simulink model "steer_by_wire"  (R2023b)
settings: Solver=VariableStepAuto  StartTime=0.0  StopTime=10.0  RelTol=1e-3
settings Model: Creator=jcm52  LastModifiedBy=jcm52

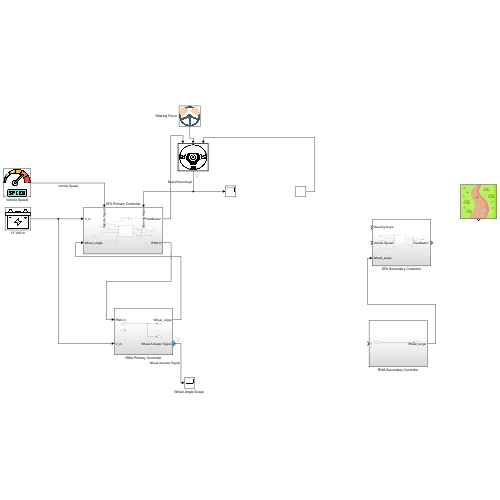
[thumbnail: Simulink's stored preview of the top-level diagram]
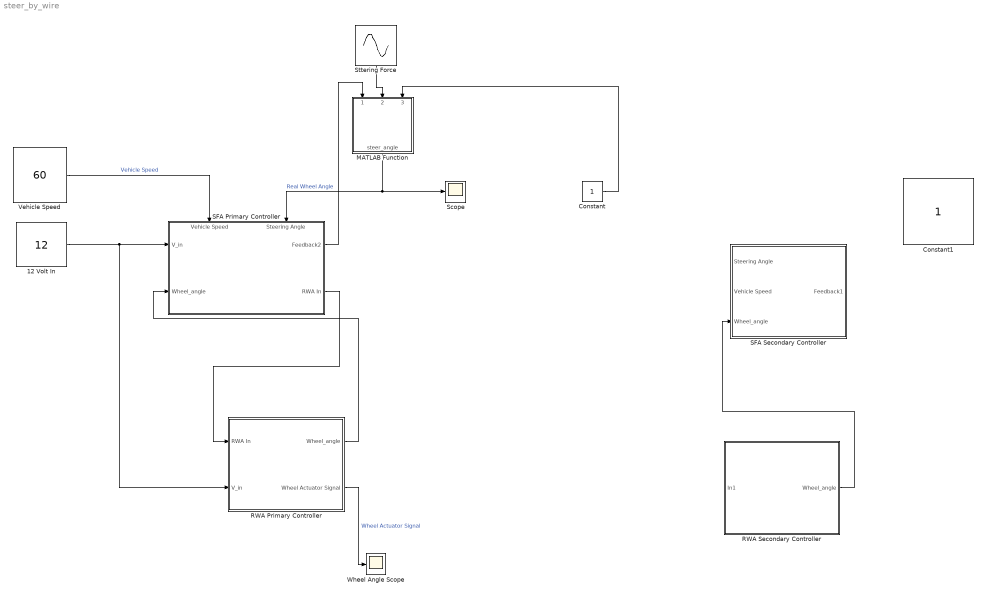
== system steer_by_wire ==
  12 Volt In : Constant  Value=12
      mask Display: image('image\free-icon-battery-3444043.png');
  Constant : Constant
  Constant1 : Constant
      mask Display: image('image\free-icon-footpath-6858832.png');
  MATLAB Function : MATLAB Function  TreatAsAtomicUnit=on
  RWA Primary Controller : Subsystem
  RWA Secondary Controller : Subsystem
  SFA Primary Controller : Subsystem
      settings: PortSchema="{\"entries\":[{\"content\":{\"sides\":[{\"content\":{\"connectorIds\":[\"Out1\",\"Out2\"]},\"type\":\"ConnectorPlacement.EquallySpacedRectSide\",\"uuid\":\"69d6b4e8-6a6c-440e-b630-8ac486e35eae\"},{\"content\":{\"connectorIds\":[\"In3\",\"In4\"],\"side\":\"RIGHT\"},\"type\":\"ConnectorPlacement.EquallySpacedRectSide\",\"uuid\":\"56fbaa10-ad34-420d-babb-7be934bb8fcf\"},{\"content\":{\"connectorIds\":[\"In1\",\"In2\"],\"side\":\"TOP\"},\"type\":\"ConnectorPlacement.EquallySpacedRectSide\",\"uuid\":\"184d897f-af35-4327-bbad-019fb4f06789\"},{\"content\":{\"side\":\"BOTTOM\"},\"type\":\"ConnectorPlacement.EquallySpacedRectSide\",\"uuid\":\"33f7de2b-e358-4395-9aa5-bc9b031e2917\"}]},\"type\":\"ConnectorPlacement.EquallySpacedConnector\",\"uuid\":\"8508fc02-ca2d-4db9-a320-47449abdf9d8\"}],\"packageUris\":[\"http://schema.mathworks.com/mf0/Connector/R2020b\"],\"version\":\"1.0\"}"
  SFA Secondary Controller : Subsystem
  Scope : Scope
  Sttering Force : Sin  Amplitude=180  SampleTime=0
      mask Display: image('image\free-icon-steering-wheel-2297514.png');
  Vehicle Speed : Constant  Value=60
      mask Display: image('image\free-icon-speed-1455318.png');
  "Wheel Angle Scope " : Scope
  wires:
  MATLAB Function/1(steer_angle) -> SFA Primary Controller/1(Steering Angle), Scope/1  "Real Wheel Angle"
  Sttering Force/1 -> MATLAB Function/2(driver_force)
  SFA Primary Controller/1("Feedback2 ") -> MATLAB Function/1(feedback1)
  Vehicle Speed/1 -> SFA Primary Controller/2(Vehicle Speed)  "Vehicle Speed"
  RWA Secondary Controller/1(Wheel_angle) -> SFA Secondary Controller/3(Wheel_angle)
  RWA Primary Controller/1(Wheel_angle) -> SFA Primary Controller/4(Wheel_angle)
  RWA Primary Controller/2(Wheel Actuator Signal) -> "Wheel Angle Scope "/1  "Wheel Actuator Signal"
  12 Volt In/1 -> RWA Primary Controller/2(V_in), SFA Primary Controller/3(V_in)
  SFA Primary Controller/2(RWA In) -> RWA Primary Controller/1(RWA In)
  Constant/1 -> MATLAB Function/3(feedback2)

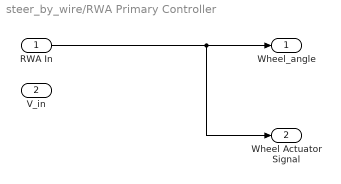
== system steer_by_wire/RWA Primary Controller ==
  RWA In : Inport
  V_in : Inport  Port=2
  Wheel_angle : Outport
  Wheel Actuator Signal : Outport  Port=2
  wires:
  RWA In/1 -> Wheel Actuator Signal/1, Wheel_angle/1

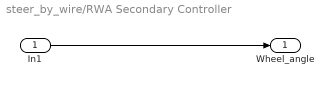
== system steer_by_wire/RWA Secondary Controller ==
  In1 : Inport
  Wheel_angle : Outport
  wires:
  In1/1 -> Wheel_angle/1

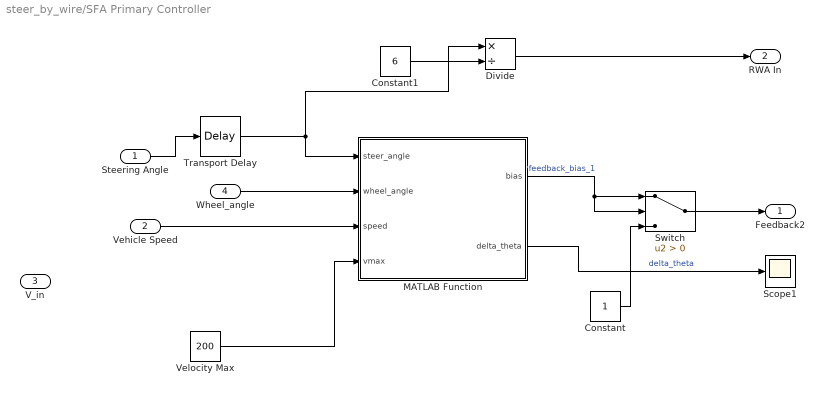
== system steer_by_wire/SFA Primary Controller ==
  Steering Angle : Inport
  Vehicle Speed : Inport  Port=2
  V_in : Inport  Port=3
  Wheel_angle : Inport  Port=4
  Constant : Constant
  Constant1 : Constant  Value=6
  Divide : Product  Inputs=*/
  MATLAB Function : MATLAB Function  TreatAsAtomicUnit=on
  Scope1 : Scope
  Switch : Switch  Criteria=u2 > Threshold  SaturateOnIntegerOverflow=off  InputSameDT=off
  Transport Delay : TransportDelay  DelayTime=0.1
  Velocity Max : Constant  Value=200
  "Feedback2 " : Outport
  RWA In : Outport  Port=2
  wires:
  Constant/1 -> Switch/3
  Switch/1 -> "Feedback2 "/1
  Steering Angle/1 -> Transport Delay/1
  Vehicle Speed/1 -> MATLAB Function/3(speed)
  Wheel_angle/1 -> MATLAB Function/2(wheel_angle)
  Velocity Max/1 -> MATLAB Function/4(vmax)
  MATLAB Function/1(bias) -> Switch/1, Switch/2  "feedback_bias_1"
  Constant1/1 -> Divide/2
  Divide/1 -> RWA In/1
  MATLAB Function/2(delta_theta) -> Scope1/1  "delta_theta"
  Transport Delay/1 -> MATLAB Function/1(steer_angle), Divide/1

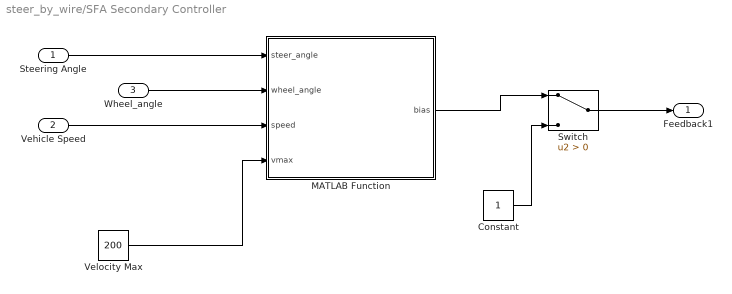
== system steer_by_wire/SFA Secondary Controller ==
  Steering Angle : Inport
  Vehicle Speed : Inport  Port=2
  Wheel_angle : Inport  Port=3
  Constant : Constant
  MATLAB Function : MATLAB Function  TreatAsAtomicUnit=on
  Switch : Switch  Criteria=u2 > Threshold  SaturateOnIntegerOverflow=off  InputSameDT=off
  Velocity Max : Constant  Value=200
  "Feedback1 " : Outport
  wires:
  Constant/1 -> Switch/3
  Switch/1 -> "Feedback1 "/1
  Steering Angle/1 -> MATLAB Function/1(steer_angle)
  Vehicle Speed/1 -> MATLAB Function/3(speed)
  Wheel_angle/1 -> MATLAB Function/2(wheel_angle)
  Velocity Max/1 -> MATLAB Function/4(vmax)
  MATLAB Function/1(bias) -> Switch/1

== matlab function steer_by_wire/SFA Secondary Controller/MATLAB Function ==
  data: steer_angle input; bias output; wheel_angle input; speed input; vmax input
function bias = calculateBias(steer_angle, wheel_angle, speed, vmax)
    % 매개변수 설정
    R = 6;               % 스티어링 비율
    alpha = 0.8;         % 속도에 따른 피드백 감소율
    K_t = 0.5;           % 조향 강성 계수

    % 각도 제한 조건 설정
    if abs(steer_angle) > 180 || abs(wheel_angle) > 30
        bias = 0;  % 각도가 제한 범위를 벗어나면 0 반환
        return;     % 함수 종료
    end

    % 각도 오차 계산
    delta_theta = steer_angle - R * wheel_angle;

    % 속도에 따른 피드백 감소 계수 계산
    beta = 1 - alpha * (speed / vmax);

    % 피드백 바이어스 계산
    bias = beta * K_t * delta_theta;
end

== matlab function steer_by_wire/MATLAB Function ==
  data: steer_angle output; feedback1 input; driver_force input; feedback2 input
function steer_angle = fcn(feedback1,driver_force,feedback2)


tmp = driver_force*feedback1*feedback2;

steer_angle = tmp;

== matlab function steer_by_wire/SFA Primary Controller/MATLAB Function ==
  data: steer_angle input; bias output; wheel_angle input; speed input; vmax input; delta_theta output
function [bias,delta_theta] = calculateBias(steer_angle, wheel_angle, speed, vmax)
    % 매개변수 설정
    R = 6;               % 스티어링 비율
    alpha = 0.8;         % 속도에 따른 피드백 감소율
    K_t = 0.5;           % 조향 강성 계수
    
    % 각도 제한 조건 설정
    if abs(steer_angle) > 180 || abs(wheel_angle) > 30
        
        bias = 0;  % 각도가 제한 범위를 벗어나면 0 반환
        delta_theta=0;
        return;     % 함수 종료
    end
    % 각도 오차 계산
    delta_theta = steer_angle - R * wheel_angle;

    % 속도에 따른 피드백 감소 계수 계산
    beta = 1 - alpha * (speed / vmax);

    % 피드백 바이어스 계산
    bias = (beta * K_t * delta_theta);
end
